simulink model "model"  (R2023a)
settings: Solver=VariableStepAuto  StartTime=0.0  StopTime=Tsim  RelTol=1e-3
values from neighbouring files (symbols this model uses):
  omega_u = 1    [Zadatak1_b.m]    (also in Zadatak1_c.m; Zadatak1_d.m; Zadatak1_e.m; Zadatak2_a.m)
  Um = 10    [Zadatak1_b.m]    (also in Zadatak1_c.m = 2; Zadatak1_d.m = 4; Zadatak1_e.m = 3; Zadatak2_a.m = 3)
  value = i    [Zadatak2_a.m]    (also in Zadatak2_b.m; Zadatak2_c.m)
  xa = 3    [Zadatak1_b.m]    (also in Zadatak1_c.m = 1.5; Zadatak1_d.m; Zadatak1_e.m; Zadatak2_a.m)
undefined symbols (not defined in the file or in its folder): den, num
settings Model: Creator=Korisnik  LastModifiedBy=Enio
settings SolverCC: AlgebraicLoopSolver=TrustRegion
settings ModelReferenceCC: EnableRefExpFcnMdlSchedulingChecks=on
settings RTWCC: DLArmComputeVersion=19.05

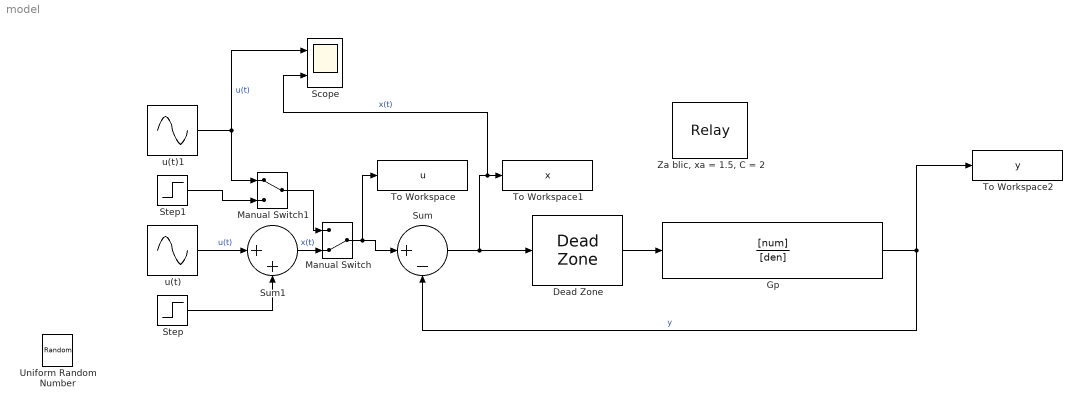
== system model ==
  Dead Zone : DeadZone  LowerValue=-xa  UpperValue=xa
  Gp : TransferFcn  Numerator=[num]  Denominator=[den]
  Manual Switch : ManualSwitch  CurrentSetting=0
  Manual Switch1 : ManualSwitch
  Scope : Scope  NumInputPorts=2
  Step : Step  After=value  SampleTime=0
  Step1 : Step  After=value  SampleTime=0
  Sum : Sum  Inputs=|+-
  Sum1 : Sum  Inputs=|++
  To Workspace : ToWorkspace  VariableName=u  SampleTime=-1
  To Workspace1 : ToWorkspace  VariableName=x  SampleTime=-1
  To Workspace2 : ToWorkspace  VariableName=y  SampleTime=-1
  Uniform Random Number : UniformRandomNumber  SampleTime=0.1
  "Za blic, xa = 1.5, C = 2" : Relay  OnSwitchValue=1.5  OffSwitchValue=-1.5  OnOutputValue=2  OffOutputValue=-2
  u(t) : Sin  Amplitude=Um  Frequency=omega_u  SampleTime=0
  u(t)1 : Sin  Amplitude=Um  Frequency=omega_u  SampleTime=0
  wires:
  Gp/1 -> Sum/2, To Workspace2/1  "y"
  Sum/1 -> Dead Zone/1, Scope/2, To Workspace1/1  "x(t)"
  u(t)/1 -> Sum1/1  "u(t)"
  Step/1 -> Sum1/2
  Manual Switch/1 -> To Workspace/1, Sum/1
  Sum1/1 -> Manual Switch/2  "x(t)"
  u(t)1/1 -> Manual Switch1/1, Scope/1  "u(t)"
  Dead Zone/1 -> Gp/1
  Manual Switch1/1 -> Manual Switch/1
  Step1/1 -> Manual Switch1/2
